simulink model "battery_sim"  (R2022a)
settings: Solver=VariableStepAuto  StartTime=0.0  StopTime=4000  RelTol=1e-3
values from neighbouring files (symbols this model uses):
  T_AMB = 298.0    [battery.sldd]    (also in simulation_parameters.m = 298)
settings Model: DataDictionary=battery.sldd  Creator=Cristobal  LastModifiedBy=Cristobal
settings SFSimCC: SimTargetLang=C++  GPUAcceleration=on  SimDLTargetLibrary=cudnn

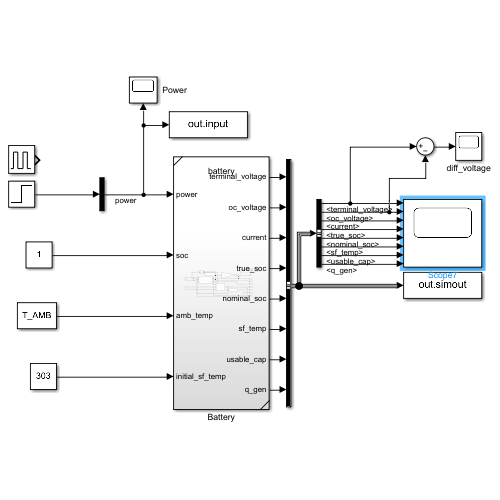
[thumbnail: Simulink's stored preview of the top-level diagram]
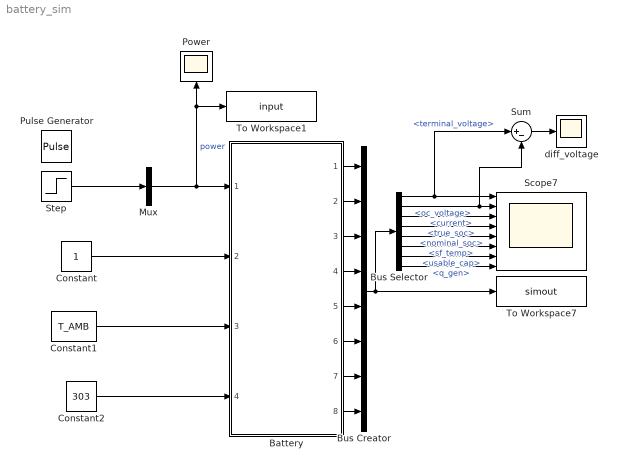
== system battery_sim ==
  Battery : Subsystem  ReferencedSubsystem=battery
  Bus Creator : BusCreator  Inputs=8
  Bus Selector : BusSelector  OutputSignals=terminal_voltage,oc_voltage,current,true_soc,nominal_soc,sf_temp,usable_cap,q_gen
  Constant : Constant
  Constant1 : Constant  Value=T_AMB
  Constant2 : Constant  Value=303
  Mux : Mux  Inputs=1
  Power : Scope
  Pulse Generator : DiscretePulseGenerator  PulseType=Time based  Amplitude=1e-1  Period=300  PulseWidth=50
  Scope7 : Scope  NumInputPorts=8
  Step : Step  Time=0  After=16  SampleTime=0
  Sum : Sum  Inputs=|+-
  To Workspace1 : ToWorkspace  VariableName=input  SaveFormat=Timeseries  SampleTime=-1
  To Workspace7 : ToWorkspace  VariableName=simout  SaveFormat=Timeseries  SampleTime=-1
  diff_voltage : Scope
  wires:
  Constant/1 -> Battery/2
  Constant1/1 -> Battery/3
  Bus Creator/1 -> Bus Selector/1, To Workspace7/1
  Battery/3 -> Bus Creator/3
  Battery/4 -> Bus Creator/4
  Battery/5 -> Bus Creator/5
  Battery/6 -> Bus Creator/6
  Battery/7 -> Bus Creator/7
  Battery/1 -> Bus Creator/1
  Battery/2 -> Bus Creator/2
  Bus Selector/1 -> Sum/1, Scope7/1  "<terminal_voltage>"
  Bus Selector/2 -> Sum/2, Scope7/2  "<oc_voltage>"
  Bus Selector/3 -> Scope7/3  "<current>"
  Bus Selector/4 -> Scope7/4  "<true_soc>"
  Bus Selector/5 -> Scope7/5  "<nominal_soc>"
  Bus Selector/6 -> Scope7/6  "<sf_temp>"
  Bus Selector/7 -> Scope7/7  "<usable_cap>"
  Battery/8 -> Bus Creator/8
  Mux/1 -> To Workspace1/1, Power/1, Battery/1  "power"
  Sum/1 -> diff_voltage/1
  Constant2/1 -> Battery/4
  Bus Selector/8 -> Scope7/8  "<q_gen>"
  Step/1 -> Mux/1
